simulink model "DC_Motor_BrakeMode_Ideal_WithGearbox"  (R2018a)
settings: Solver=VariableStepAuto  StartTime=0.0  StopTime=10.0  FixedStep=1e-5  RelTol=1e-3
settings Model: Creator=Thomas  LastModifiedBy=Thomas

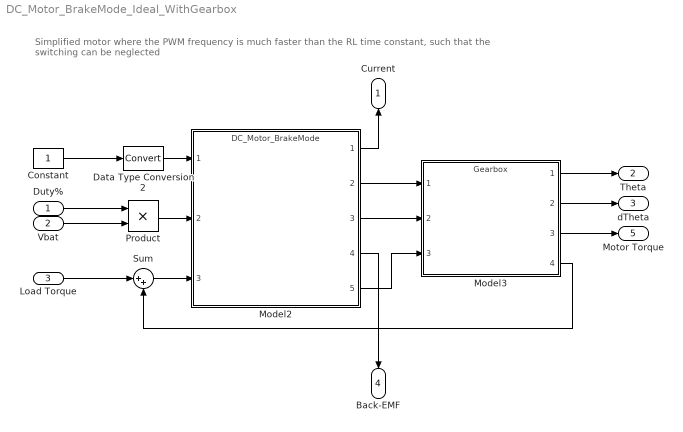
== system DC_Motor_BrakeMode_Ideal_WithGearbox ==
  note: Simplified motor where the PWM frequency is much faster than the RL time constant, such that the switching can be neglected
  Duty% : Inport  OutDataTypeStr=double
  Vbat : Inport  Port=2  OutDataTypeStr=double
  Load Torque : Inport  Port=3  OutDataTypeStr=double
  Constant : Constant
  Data Type Conversion2 : DataTypeConversion  RndMeth=Round
  Model2 : ModelReference  ModelNameDialog=DC_Motor_BrakeMode  SimulationMode=Normal  ModelReferenceVersion=1.33
  Model3 : ModelReference  ModelNameDialog=Gearbox  SimulationMode=Normal  ModelReferenceVersion=1.7
  Product : Product
  Sum : Sum  Inputs=|++
  Current : Outport
  Theta : Outport  Port=2
  dTheta : Outport  Port=3
  Back-EMF : Outport  Port=4
  Motor Torque : Outport  Port=5
  wires:
  Model2/2 -> Model3/1
  Model2/3 -> Model3/2
  Model2/1 -> Current/1
  Data Type Conversion2/1 -> Model2/1
  Duty%/1 -> Product/1
  Constant/1 -> Data Type Conversion2/1
  Vbat/1 -> Product/2
  Product/1 -> Model2/2
  Model3/1 -> Theta/1
  Model3/2 -> dTheta/1
  Model2/5 -> Model3/3
  Load Torque/1 -> Sum/1
  Model3/4 -> Sum/2
  Sum/1 -> Model2/3
  Model3/3 -> Motor Torque/1
  Model2/4 -> Back-EMF/1
